simulink model "Lab05"  (R2024b)
settings: Solver=ode8  StartTime=0.0  StopTime=tf  FixedStep=0.025  RelTol=1e-3
values from neighbouring files (symbols this model uses):
  I = diag(Iv)    [initLab5.m]
  invI = inv(I)    [initLab5.m]
  w0 = [0.45; 0.52; 0.55]    [initLab5.m]
undefined symbols (not defined in the file or in its folder): IC
libraries: matrix_library x1
(part 3 of 4)

== system Lab05/EuleroCompletoCheGiraMaAlgebrico1/A313 ==
  In1 : Inport
  Cos : Trigonometry  Operator=cos
  Cos1 : Trigonometry  Operator=cos
  Cos2 : Trigonometry  Operator=cos
  Demux : Demux  Outputs=3
  Gain : Gain  Gain=-1
  Matrix Concatenate : Concatenate  NumInputs=3  Mode=Multidimensional array
  Matrix Concatenate1 : Concatenate  NumInputs=3  Mode=Multidimensional array
  Matrix Concatenate3 : Concatenate  NumInputs=3  Mode=Multidimensional array  ConcatenateDimension=2
  Matrix Concatenate4 : Concatenate  NumInputs=3  Mode=Multidimensional array
  Product{1,3,5..6,8,10..12} (8 alike) : Product
  Product{2,4,7,9} (4 alike) : Product  Inputs=3
  Sin : Trigonometry
  Sin1 : Trigonometry
  Sin2 : Trigonometry
  Subtract : Sum  Inputs=+-
  Subtract1 : Sum  Inputs=--
  Subtract2 : Sum
  Subtract3 : Sum  Inputs=-+
  Out1 : Outport
  wires:
  In1/1 -> Demux/1
  [cosTheta] -> Product2/3
  Product7/1 -> Subtract2/2
  [sinTheta] -> Product11/2
  [sinPhi] -> Product8/2
  Sin/1 -> [sinPhi]
  [cosTheta] -> Product4/3
  [sinPhi] -> Product2/2
  [sinTheta] -> Product10/2
  Product5/1 -> Matrix Concatenate/3
  [cosPsi] -> Product6/1
  Demux/3 -> Sin2/1, Cos2/1
  Product9/1 -> Subtract3/2
  [cosTheta] -> Matrix Concatenate1/3
  Matrix Concatenate1/1 -> Matrix Concatenate3/3
  [sinPsi] -> Product11/1
  Product2/1 -> Subtract/2
  [sinPhi] -> Product4/2
  Subtract2/1 -> Matrix Concatenate4/1
  Matrix Concatenate4/1 -> Matrix Concatenate3/2
  [cosPsi] -> Product12/1
  Cos2/1 -> [cosPsi]
  Product10/1 -> Gain/1
  [sinPsi] -> Product2/1
  [sinPsi] -> Product8/1
  Sin2/1 -> [sinPsi]
  [cosTheta] -> Product7/3
  Subtract/1 -> Matrix Concatenate/1
  [cosPhi] -> Product10/1
  Subtract1/1 -> Matrix Concatenate/2
  Subtract3/1 -> Matrix Concatenate4/2
  Demux/2 -> Sin1/1, Cos1/1
  [cosTheta] -> Product9/3
  Product8/1 -> Subtract3/1
  [cosPhi] -> Product9/2
  [cosPsi] -> Product9/1
  Gain/1 -> Matrix Concatenate4/3
  [cosPsi] -> Product4/1
  Product11/1 -> Matrix Concatenate1/1
  Product1/1 -> Subtract/1
  [cosPhi] -> Product1/2
  [sinTheta] -> Product12/2
  [cosPhi] -> Product7/2
  [sinPhi] -> Product6/2
  Product6/1 -> Subtract2/1
  Demux/1 -> Sin/1, Cos/1
  [cosPsi] -> Product1/1
  [sinPsi] -> Product7/1
  Cos1/1 -> [cosTheta]
  Sin1/1 -> [sinTheta]
  [sinTheta] -> Product5/2
  [sinPsi] -> Product3/1
  Product12/1 -> Matrix Concatenate1/2
  [sinPhi] -> Product5/1
  Product3/1 -> Subtract1/1
  Product4/1 -> Subtract1/2
  [cosPhi] -> Product3/2
  Matrix Concatenate/1 -> Matrix Concatenate3/1
  Cos/1 -> [cosPhi]
  Matrix Concatenate3/1 -> Out1/1

== system Lab05/EuleroCompletoCheGiraMaAlgebrico2/312 ==
  In1 : Inport
  In2 : Inport  Port=2
  In3 : Inport  Port=3
  Cos1 : Trigonometry  Operator=cos
  Cos2 : Trigonometry  Operator=cos
  Demux : Demux  Outputs=3
  Demux1 : Demux  Outputs=3
  Divide1 : Product  Inputs=*/
  IC : InitialCondition  Value=IC.angles
  Integrator1 : Integrator  ExternalReset=either  InitialConditionSource=external  WrapState=on  WrappedStateUpperValue=2*pi  WrappedStateLowerValue=0
  Integrator2 : Integrator  ExternalReset=either  InitialConditionSource=external  WrapState=on
  Integrator3 : Integrator  ExternalReset=either  InitialConditionSource=external  WrapState=on  WrappedStateUpperValue=2*pi  WrappedStateLowerValue=0
  Mux : Mux  Inputs=3
  Product{1..7} (7 alike) : Product
  Sin : Trigonometry
  Subtract : Sum  Inputs=+-
  Subtract1 : Sum
  Subtract2 : Sum  Inputs=+-
  Subtract3 : Sum  Inputs=+-
  Tan : Trigonometry  Operator=tan
  Out1 : Outport
  wires:
  Product6/1 -> Subtract3/2
  Product5/1 -> Subtract3/1
  Product4/1 -> Subtract1/2
  Integrator3/1 -> [theta3]
  [wz] -> Product5/1
  Mux/1 -> Out1/1
  Product7/1 -> Subtract2/2
  Cos1/1 -> [cosPsi]
  [theta3] -> Sin/1, Cos1/1
  [cosPsi] -> Product1/2
  Demux/2 -> [wy]
  Tan/1 -> [tanThe]
  Product2/1 -> Subtract/2
  [wz] -> Product3/1
  [tanThe] -> Product7/2
  Cos2/1 -> [cosThe]
  [cosPsi] -> Product5/2
  Divide1/1 -> Integrator1/1
  Subtract1/1 -> Integrator2/1
  Demux/3 -> [wz]
  [theta1] -> Mux/1
  Subtract/1 -> Divide1/1
  Demux/1 -> [wx]
  Subtract2/1 -> Integrator3/1
  [theta2] -> Tan/1, Cos2/1
  [wy] -> Subtract2/1
  Integrator1/1 -> [theta1]
  Integrator2/1 -> [theta2]
  [wx] -> Product4/1
  [sinPsi] -> Product2/2
  In1/1 -> Demux/1
  Subtract3/1 -> Product7/1
  Product3/1 -> Subtract1/1
  [theta2] -> Mux/2
  [sinPsi] -> Product3/2
  [theta3] -> Mux/3
  [sinPsi] -> Product6/2
  [wx] -> Product6/1
  [wx] -> Product2/1
  [cosPsi] -> Product4/2
  [wz] -> Product1/1
  Product1/1 -> Subtract/1
  [cosThe] -> Divide1/2
  Sin/1 -> [sinPsi]
  Demux1/1 -> Integrator1/3
  Demux1/2 -> Integrator2/3
  Demux1/3 -> Integrator3/3
  In2/1 -> IC/1
  IC/1 -> Demux1/1
  In3/1 -> Integrator2/2, Integrator3/2, Integrator1/2

== system Lab05/EuleroCompletoCheGiraMaAlgebrico2/312To313 ==
  note: Important
      |
      | This system is based on the assumptions that Phi and Psi ranges between [0 and 2*pi] while Theta ranges between [0 and pi]. This is consistent with 313 singularities
  note: Input Interface
  In1 : Inport
  Acos : Trigonometry  Operator=acos
  Acos1 : Trigonometry  Operator=acos
  Atan2 : Trigonometry  Operator=atan2
  Atan3 : Trigonometry  Operator=atan2
  Cos : Trigonometry  Operator=cos
  Cos1 : Trigonometry  Operator=cos
  Cos2 : Trigonometry  Operator=cos
  Demux : Demux  Outputs=3
  Divide{,1..3} (4 alike) : Product  Inputs=*/
  Gain : Gain  Gain=-1
  Gain1 : Gain  Gain=-1
  Mux : Mux  Inputs=3
  Product{,3,8,11} (4 alike) : Product
  Product4 : Product  Inputs=3
  Product9 : Product  Inputs=3
  Sin{,1..3} (4 alike) : Trigonometry
  Subtract1 : Sum
  Subtract3 : Sum  Inputs=+-
  Out1 : Outport
  wires:
  In1/1 -> Demux/1
  Mux/1 -> Out1/1
  Sin/1 -> [sinPhi312]
  Cos/1 -> [cosPhi312]
  Demux/1 -> Sin/1, Cos/1
  Sin1/1 -> [sinTheta312]
  Demux/2 -> Sin1/1, Cos1/1
  Cos1/1 -> [cosTheta312]
  Sin2/1 -> [sinPsi312]
  Cos2/1 -> [cosPsi312]
  Demux/3 -> Sin2/1, Cos2/1
  Product/1 -> Acos1/1, [cosTheta313]
  [cosTheta312] -> Product/2
  [cosPsi312] -> Product/1
  Atan2/1 -> Mux/1
  Acos/1 -> Mux/2
  Atan3/1 -> Mux/3
  [sinPhi313] -> Atan2/1
  [cosPhi313] -> Atan2/2
  [cosTheta313] -> Acos/1
  [cosPsi313] -> Atan3/2
  [sinPsi313] -> Atan3/1
  Sin3/1 -> [sinTheta313]
  Acos1/1 -> Sin3/1
  [cosPsi312] -> Product4/1
  [sinTheta312] -> Product4/3
  Product3/1 -> Subtract1/1
  [cosPhi312] -> Product3/2
  Product4/1 -> Subtract1/2
  [sinPsi312] -> Product3/1
  [sinPhi312] -> Product4/2
  Divide/1 -> [sinPhi313]
  [sinTheta313] -> Divide/2
  Subtract1/1 -> Divide/1
  Gain/1 -> [cosPhi313]
  Divide1/1 -> Gain/1
  [sinTheta313] -> Divide1/2
  [cosPsi312] -> Product9/1
  Product9/1 -> Subtract3/2
  Subtract3/1 -> Divide1/1
  [sinPsi312] -> Product8/1
  [cosPhi312] -> Product9/2
  [sinPhi312] -> Product8/2
  [sinTheta312] -> Product9/3
  Product8/1 -> Subtract3/1
  [sinTheta313] -> Divide2/2
  Divide2/1 -> [sinPsi313]
  [sinTheta313] -> Divide3/2
  Divide3/1 -> [cosPsi313]
  Product11/1 -> Gain1/1
  [sinPsi312] -> Product11/1
  [cosTheta312] -> Product11/2
  Gain1/1 -> Divide2/1
  [sinTheta312] -> Divide3/1

== system Lab05/EuleroCompletoCheGiraMaAlgebrico2/313 ==
  note: Phi
  note: Theta
  In2 : Inport
  In1 : Inport  Port=2
  In3 : Inport  Port=3
  Cos1 : Trigonometry  Operator=cos
  Cos2 : Trigonometry
  Demux : Demux  Outputs=3
  Demux1 : Demux  Outputs=3
  Divide : Product  Inputs=/
  Divide1 : Product  Inputs=*/
  IC : InitialCondition  Value=IC.angles
  Integrator1 : Integrator  ExternalReset=either  InitialConditionSource=external  WrapState=on  WrappedStateUpperValue=2*pi  WrappedStateLowerValue=0
  Integrator2 : Integrator  ExternalReset=either  InitialConditionSource=external  InitialCondition=pi/4  WrapState=on
  Integrator3 : Integrator  ExternalReset=either  InitialConditionSource=external  WrapState=on  WrappedStateUpperValue=2*pi  WrappedStateLowerValue=0
  Mux : Mux  Inputs=3
  Product{1..7} (7 alike) : Product
  Sin : Trigonometry
  Subtract : Sum
  Subtract1 : Sum  Inputs=-+
  Subtract2 : Sum  Inputs=+-
  Subtract3 : Sum
  Tan : Trigonometry  Operator=tan
  Out1 : Outport
  wires:
  [sinThe] -> Divide1/2
  Sin/1 -> [sinPsi]
  [wx] -> Product2/1
  [theta3] -> Mux/3
  [theta2] -> Mux/2
  Product3/1 -> Subtract1/1
  In1/1 -> Demux/1
  [sinPsi] -> Product3/2
  [sinPsi] -> Product6/2
  Subtract3/1 -> Product7/1
  Product1/1 -> Subtract/1
  [wx] -> Product6/1
  [wy] -> Product1/1
  [wz] -> Subtract2/1
  Subtract2/1 -> Integrator3/1
  [theta2] -> Tan/1, Cos2/1
  [cosPsi] -> Product4/2
  Demux/1 -> [wx]
  [sinPsi] -> Product2/2
  Integrator2/1 -> [theta2]
  [wx] -> Product4/1
  Tan/1 -> Divide/1
  [cosPsi] -> Product1/2
  Divide1/1 -> Integrator1/1
  Integrator1/1 -> [theta1]
  [ctanThe] -> Product7/2
  [cosPsi] -> Product5/2
  [wy] -> Product3/1
  Product2/1 -> Subtract/2
  Demux/2 -> [wy]
  Product5/1 -> Subtract3/1
  [wy] -> Product5/1
  Integrator3/1 -> [theta3]
  Product6/1 -> Subtract3/2
  Mux/1 -> Out1/1
  Product4/1 -> Subtract1/2
  [theta3] -> Sin/1, Cos1/1
  Product7/1 -> Subtract2/2
  Cos2/1 -> [sinThe]
  Subtract1/1 -> Integrator2/1
  [theta1] -> Mux/1
  Subtract/1 -> Divide1/1
  Demux/3 -> [wz]
  Cos1/1 -> [cosPsi]
  Divide/1 -> [ctanThe]
  Demux1/3 -> Integrator3/3
  Demux1/2 -> Integrator2/3
  Demux1/1 -> Integrator1/3
  IC/1 -> Demux1/1
  In3/1 -> Integrator1/2, Integrator2/2, Integrator3/2
  In2/1 -> IC/1

== system Lab05/EuleroCompletoCheGiraMaAlgebrico2/313To1 ==
  note: Input Interface
  note: Important
      |
      | This system is based on the assumptions that Phi and Psi ranges between [0 and 2*pi] while Theta ranges between [-pi/2 and pi/2]. This is consistent with 312 singularities
  In1 : Inport
  Acos : Trigonometry  Operator=asin
  Acos1 : Trigonometry  Operator=asin
  Atan2 : Trigonometry  Operator=atan2
  Atan3 : Trigonometry  Operator=atan2
  Cos : Trigonometry  Operator=cos
  Cos1 : Trigonometry  Operator=cos
  Cos2 : Trigonometry  Operator=cos
  Demux : Demux  Outputs=3
  Divide{,1..3} (4 alike) : Product  Inputs=*/
  Gain : Gain  Gain=-1
  Gain1 : Gain  Gain=-1
  Mux : Mux  Inputs=3
  Product{,3,8,11} (4 alike) : Product
  Product4 : Product  Inputs=3
  Product9 : Product  Inputs=3
  Sin : Trigonometry
  Sin1 : Trigonometry
  Sin2 : Trigonometry
  Sin3 : Trigonometry  Operator=cos
  Subtract1 : Sum  Inputs=--
  Subtract3 : Sum  Inputs=-+
  Out1 : Outport
  wires:
  Cos/1 -> [cosPhi313]
  Sin/1 -> [sinPhi313]
  Cos1/1 -> [cosTheta313]
  Demux/3 -> Sin2/1, Cos2/1
  Demux/1 -> Sin/1, Cos/1
  Sin2/1 -> [sinPsi313]
  Sin1/1 -> [sinTheta313]
  In1/1 -> Demux/1
  Demux/2 -> Sin1/1, Cos1/1
  Cos2/1 -> [cosPsi313]
  Mux/1 -> Out1/1
  [sinTheta312] -> Acos/1
  Atan3/1 -> Mux/3
  Atan2/1 -> Mux/1
  [sinPhi312] -> Atan2/1
  [cosPhi312] -> Atan2/2
  [sinPsi312] -> Atan3/1
  [cosPsi312] -> Atan3/2
  Acos/1 -> Mux/2
  [sinTheta313] -> Product/2
  Product/1 -> Acos1/1, [sinTheta312]
  Sin3/1 -> [cosTheta312]
  [cosPsi313] -> Product/1
  Acos1/1 -> Sin3/1
  Gain/1 -> [sinPhi312]
  Divide/1 -> Gain/1
  [cosTheta312] -> Divide/2
  Product3/1 -> Subtract1/1
  [cosPhi313] -> Product3/2
  Product4/1 -> Subtract1/2
  [cosPsi313] -> Product4/1
  [sinPhi313] -> Product4/2
  Subtract1/1 -> Divide/1
  [sinPsi313] -> Product3/1
  [cosTheta313] -> Product4/3
  [cosTheta312] -> Divide1/2
  Divide1/1 -> [cosPhi312]
  [cosPsi313] -> Product9/1
  Product9/1 -> Subtract3/2
  [sinPsi313] -> Product8/1
  [sinPhi313] -> Product8/2
  Product8/1 -> Subtract3/1
  [cosTheta313] -> Product9/3
  Subtract3/1 -> Divide1/1
  [cosPhi313] -> Product9/2
  Divide2/1 -> Gain1/1
  [cosTheta312] -> Divide2/2
  Gain1/1 -> [sinPsi312]
  [sinTheta313] -> Product11/2
  Product11/1 -> Divide2/1
  [sinPsi313] -> Product11/1
  [cosTheta312] -> Divide3/2
  [cosTheta313] -> Divide3/1
  Divide3/1 -> [cosPsi312]

== system Lab05/EuleroCompletoCheGiraMaAlgebrico2/313To312 ==
  note: Input Interface
  note: Important
      |
      | This system is based on the assumptions that Phi and Psi ranges between [0 and 2*pi] while Theta ranges between [-pi/2 and pi/2]. This is consistent with 312 singularities
  In1 : Inport
  Acos : Trigonometry  Operator=asin
  Acos1 : Trigonometry  Operator=asin
  Atan2 : Trigonometry  Operator=atan2
  Atan3 : Trigonometry  Operator=atan2
  Cos : Trigonometry  Operator=cos
  Cos1 : Trigonometry  Operator=cos
  Cos2 : Trigonometry  Operator=cos
  Demux : Demux  Outputs=3
  Divide{,1..3} (4 alike) : Product  Inputs=*/
  Gain : Gain  Gain=-1
  Gain1 : Gain  Gain=-1
  Mux : Mux  Inputs=3
  Product{,3,8,11} (4 alike) : Product
  Product4 : Product  Inputs=3
  Product9 : Product  Inputs=3
  Sin : Trigonometry
  Sin1 : Trigonometry
  Sin2 : Trigonometry
  Sin3 : Trigonometry  Operator=cos
  Subtract1 : Sum  Inputs=--
  Subtract3 : Sum  Inputs=-+
  Out1 : Outport
  wires:
  Cos/1 -> [cosPhi313]
  Sin/1 -> [sinPhi313]
  Cos1/1 -> [cosTheta313]
  Demux/3 -> Sin2/1, Cos2/1
  Demux/1 -> Sin/1, Cos/1
  Sin2/1 -> [sinPsi313]
  Sin1/1 -> [sinTheta313]
  In1/1 -> Demux/1
  Demux/2 -> Sin1/1, Cos1/1
  Cos2/1 -> [cosPsi313]
  Mux/1 -> Out1/1
  [sinTheta312] -> Acos/1
  Atan3/1 -> Mux/3
  Atan2/1 -> Mux/1
  [sinPhi312] -> Atan2/1
  [cosPhi312] -> Atan2/2
  [sinPsi312] -> Atan3/1
  [cosPsi312] -> Atan3/2
  Acos/1 -> Mux/2
  [sinTheta313] -> Product/2
  Product/1 -> Acos1/1, [sinTheta312]
  Sin3/1 -> [cosTheta312]
  [cosPsi313] -> Product/1
  Acos1/1 -> Sin3/1
  Gain/1 -> [sinPhi312]
  Divide/1 -> Gain/1
  [cosTheta312] -> Divide/2
  Product3/1 -> Subtract1/1
  [cosPhi313] -> Product3/2
  Product4/1 -> Subtract1/2
  [cosPsi313] -> Product4/1
  [sinPhi313] -> Product4/2
  Subtract1/1 -> Divide/1
  [sinPsi313] -> Product3/1
  [cosTheta313] -> Product4/3
  [cosTheta312] -> Divide1/2
  Divide1/1 -> [cosPhi312]
  [cosPsi313] -> Product9/1
  Product9/1 -> Subtract3/2
  [sinPsi313] -> Product8/1
  [sinPhi313] -> Product8/2
  Product8/1 -> Subtract3/1
  [cosTheta313] -> Product9/3
  Subtract3/1 -> Divide1/1
  [cosPhi313] -> Product9/2
  Divide2/1 -> Gain1/1
  [cosTheta312] -> Divide2/2
  Gain1/1 -> [sinPsi312]
  [sinTheta313] -> Product11/2
  Product11/1 -> Divide2/1
  [sinPsi313] -> Product11/1
  [cosTheta312] -> Divide3/2
  [cosTheta313] -> Divide3/1
  Divide3/1 -> [cosPsi312]

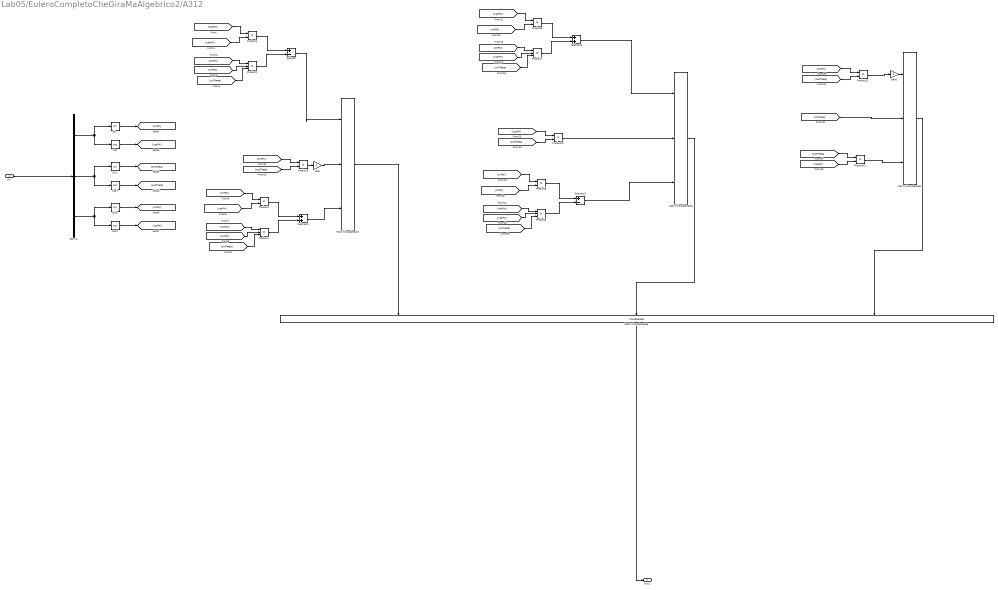
== system Lab05/EuleroCompletoCheGiraMaAlgebrico2/A312 ==
  In1 : Inport
  Cos : Trigonometry  Operator=cos
  Cos1 : Trigonometry  Operator=cos
  Cos2 : Trigonometry  Operator=cos
  Demux : Demux  Outputs=3
  Gain : Gain  Gain=-1
  Gain1 : Gain  Gain=-1
  Matrix Concatenate : Concatenate  NumInputs=3  Mode=Multidimensional array
  Matrix Concatenate1 : Concatenate  NumInputs=3  Mode=Multidimensional array
  Matrix Concatenate3 : Concatenate  NumInputs=3  Mode=Multidimensional array  ConcatenateDimension=2
  Matrix Concatenate4 : Concatenate  NumInputs=3  Mode=Multidimensional array
  Product{1,3,5..6,8,10..12} (8 alike) : Product
  Product{2,4,7,9} (4 alike) : Product  Inputs=3
  Sin : Trigonometry
  Sin1 : Trigonometry
  Sin2 : Trigonometry
  Subtract : Sum  Inputs=+-
  Subtract1 : Sum
  Subtract2 : Sum
  Subtract3 : Sum  Inputs=+-
  Out1 : Outport
  wires:
  In1/1 -> Demux/1
  [sinTheta] -> Product2/3
  Product7/1 -> Subtract2/2
  [cosTheta] -> Product11/2
  [sinPhi] -> Product8/2
  Sin/1 -> [sinPhi]
  [sinPhi] -> Product2/2
  [cosTheta] -> Product10/2
  [cosPsi] -> Product6/1
  Demux/3 -> Sin2/1, Cos2/1
  Product9/1 -> Subtract3/2
  [sinTheta] -> Matrix Concatenate1/2
  Matrix Concatenate1/1 -> Matrix Concatenate3/3
  [sinPsi] -> Product11/1
  Product2/1 -> Subtract/2
  Subtract2/1 -> Matrix Concatenate4/1
  Matrix Concatenate4/1 -> Matrix Concatenate3/2
  [cosTheta] -> Product12/1
  Cos2/1 -> [cosPsi]
  [sinPsi] -> Product2/1
  [sinPsi] -> Product8/1
  Sin2/1 -> [sinPsi]
  [sinTheta] -> Product7/3
  Subtract/1 -> Matrix Concatenate/1
  [cosPhi] -> Product10/1
  Demux/2 -> Sin1/1, Cos1/1
  [sinTheta] -> Product9/3
  Product8/1 -> Subtract3/1
  [cosPhi] -> Product9/2
  [cosPsi] -> Product9/1
  Product11/1 -> Gain1/1
  Product1/1 -> Subtract/1
  [cosPhi] -> Product1/2
  [cosPsi] -> Product12/2
  [cosPhi] -> Product7/2
  [sinPhi] -> Product6/2
  Product6/1 -> Subtract2/1
  Demux/1 -> Sin/1, Cos/1
  [cosPsi] -> Product1/1
  [sinPsi] -> Product7/1
  Cos1/1 -> [cosTheta]
  Sin1/1 -> [sinTheta]
  Product12/1 -> Matrix Concatenate1/3
  Matrix Concatenate/1 -> Matrix Concatenate3/1
  Cos/1 -> [cosPhi]
  Matrix Concatenate3/1 -> Out1/1
  Gain1/1 -> Matrix Concatenate1/1
  Product10/1 -> Matrix Concatenate4/2
  Subtract3/1 -> Matrix Concatenate4/3
  [cosPsi] -> Product4/1
  Product4/1 -> Subtract1/2
  [cosPhi] -> Product3/2
  Product3/1 -> Subtract1/1
  [sinPsi] -> Product3/1
  [sinPhi] -> Product4/2
  [sinTheta] -> Product4/3
  [sinPhi] -> Product5/1
  [cosTheta] -> Product5/2
  Product5/1 -> Gain/1
  Subtract1/1 -> Matrix Concatenate/3
  Gain/1 -> Matrix Concatenate/2

== system Lab05/EuleroCompletoCheGiraMaAlgebrico2/A313 ==
  In1 : Inport
  Cos : Trigonometry  Operator=cos
  Cos1 : Trigonometry  Operator=cos
  Cos2 : Trigonometry  Operator=cos
  Demux : Demux  Outputs=3
  Gain : Gain  Gain=-1
  Matrix Concatenate : Concatenate  NumInputs=3  Mode=Multidimensional array
  Matrix Concatenate1 : Concatenate  NumInputs=3  Mode=Multidimensional array
  Matrix Concatenate3 : Concatenate  NumInputs=3  Mode=Multidimensional array  ConcatenateDimension=2
  Matrix Concatenate4 : Concatenate  NumInputs=3  Mode=Multidimensional array
  Product{1,3,5..6,8,10..12} (8 alike) : Product
  Product{2,4,7,9} (4 alike) : Product  Inputs=3
  Sin : Trigonometry
  Sin1 : Trigonometry
  Sin2 : Trigonometry
  Subtract : Sum  Inputs=+-
  Subtract1 : Sum  Inputs=--
  Subtract2 : Sum
  Subtract3 : Sum  Inputs=-+
  Out1 : Outport
  wires:
  In1/1 -> Demux/1
  [cosTheta] -> Product2/3
  Product7/1 -> Subtract2/2
  [sinTheta] -> Product11/2
  [sinPhi] -> Product8/2
  Sin/1 -> [sinPhi]
  [cosTheta] -> Product4/3
  [sinPhi] -> Product2/2
  [sinTheta] -> Product10/2
  Product5/1 -> Matrix Concatenate/3
  [cosPsi] -> Product6/1
  Demux/3 -> Sin2/1, Cos2/1
  Product9/1 -> Subtract3/2
  [cosTheta] -> Matrix Concatenate1/3
  Matrix Concatenate1/1 -> Matrix Concatenate3/3
  [sinPsi] -> Product11/1
  Product2/1 -> Subtract/2
  [sinPhi] -> Product4/2
  Subtract2/1 -> Matrix Concatenate4/1
  Matrix Concatenate4/1 -> Matrix Concatenate3/2
  [cosPsi] -> Product12/1
  Cos2/1 -> [cosPsi]
  Product10/1 -> Gain/1
  [sinPsi] -> Product2/1
  [sinPsi] -> Product8/1
  Sin2/1 -> [sinPsi]
  [cosTheta] -> Product7/3
  Subtract/1 -> Matrix Concatenate/1
  [cosPhi] -> Product10/1
  Subtract1/1 -> Matrix Concatenate/2
  Subtract3/1 -> Matrix Concatenate4/2
  Demux/2 -> Sin1/1, Cos1/1
  [cosTheta] -> Product9/3
  Product8/1 -> Subtract3/1
  [cosPhi] -> Product9/2
  [cosPsi] -> Product9/1
  Gain/1 -> Matrix Concatenate4/3
  [cosPsi] -> Product4/1
  Product11/1 -> Matrix Concatenate1/1
  Product1/1 -> Subtract/1
  [cosPhi] -> Product1/2
  [sinTheta] -> Product12/2
  [cosPhi] -> Product7/2
  [sinPhi] -> Product6/2
  Product6/1 -> Subtract2/1
  Demux/1 -> Sin/1, Cos/1
  [cosPsi] -> Product1/1
  [sinPsi] -> Product7/1
  Cos1/1 -> [cosTheta]
  Sin1/1 -> [sinTheta]
  [sinTheta] -> Product5/2
  [sinPsi] -> Product3/1
  Product12/1 -> Matrix Concatenate1/2
  [sinPhi] -> Product5/1
  Product3/1 -> Subtract1/1
  Product4/1 -> Subtract1/2
  [cosPhi] -> Product3/2
  Matrix Concatenate/1 -> Matrix Concatenate3/1
  Cos/1 -> [cosPhi]
  Matrix Concatenate3/1 -> Out1/1

== system Lab05/EuleroCompletoCheGiraMale/312 ==
  In1 : Inport
  In2 : Inport  Port=2
  Enable : EnablePort  StatesWhenEnabling=reset
  Cos1 : Trigonometry  Operator=cos
  Cos2 : Trigonometry  Operator=cos
  Demux : Demux  Outputs=3
  Demux1 : Demux  Outputs=3
  Divide1 : Product  Inputs=*/
  IC : InitialCondition  Value=IC.angles
  Integrator1 : Integrator  InitialConditionSource=external  WrapState=on  WrappedStateUpperValue=2*pi  WrappedStateLowerValue=0
  Integrator2 : Integrator  InitialConditionSource=external  WrapState=on
  Integrator3 : Integrator  InitialConditionSource=external  WrapState=on  WrappedStateUpperValue=2*pi  WrappedStateLowerValue=0
  Mux : Mux  Inputs=3
  Product{1..7} (7 alike) : Product
  Sin : Trigonometry
  Subtract : Sum  Inputs=+-
  Subtract1 : Sum
  Subtract2 : Sum  Inputs=+-
  Subtract3 : Sum  Inputs=+-
  Tan : Trigonometry  Operator=tan
  Out1 : Outport
  wires:
  Product6/1 -> Subtract3/2
  Product5/1 -> Subtract3/1
  Product4/1 -> Subtract1/2
  Integrator3/1 -> [theta3]
  [wz] -> Product5/1
  Mux/1 -> Out1/1
  Product7/1 -> Subtract2/2
  Cos1/1 -> [cosPsi]
  [theta3] -> Sin/1, Cos1/1
  [cosPsi] -> Product1/2
  Demux/2 -> [wy]
  Tan/1 -> [tanThe]
  Product2/1 -> Subtract/2
  [wz] -> Product3/1
  [tanThe] -> Product7/2
  Cos2/1 -> [cosThe]
  [cosPsi] -> Product5/2
  Divide1/1 -> Integrator1/1
  Subtract1/1 -> Integrator2/1
  Demux/3 -> [wz]
  [theta1] -> Mux/1
  Subtract/1 -> Divide1/1
  Demux/1 -> [wx]
  Subtract2/1 -> Integrator3/1
  [theta2] -> Tan/1, Cos2/1
  [wy] -> Subtract2/1
  Integrator1/1 -> [theta1]
  Integrator2/1 -> [theta2]
  [wx] -> Product4/1
  [sinPsi] -> Product2/2
  In1/1 -> Demux/1
  Subtract3/1 -> Product7/1
  Product3/1 -> Subtract1/1
  [theta2] -> Mux/2
  [sinPsi] -> Product3/2
  [theta3] -> Mux/3
  [sinPsi] -> Product6/2
  [wx] -> Product6/1
  [wx] -> Product2/1
  [cosPsi] -> Product4/2
  [wz] -> Product1/1
  Product1/1 -> Subtract/1
  [cosThe] -> Divide1/2
  Sin/1 -> [sinPsi]
  Demux1/1 -> Integrator1/2
  Demux1/2 -> Integrator2/2
  Demux1/3 -> Integrator3/2
  In2/1 -> IC/1
  IC/1 -> Demux1/1

== system Lab05/EuleroCompletoCheGiraMale/312To313 ==
  note: Important
      |
      | This system is based on the assumptions that Phi and Psi ranges between [0 and 2*pi] while Theta ranges between [0 and pi]. This is consistent with 313 singularities
  note: Input Interface
  In1 : Inport
  Acos : Trigonometry  Operator=acos
  Acos1 : Trigonometry  Operator=acos
  Atan2 : Trigonometry  Operator=atan2
  Atan3 : Trigonometry  Operator=atan2
  Cos : Trigonometry  Operator=cos
  Cos1 : Trigonometry  Operator=cos
  Cos2 : Trigonometry  Operator=cos
  Demux : Demux  Outputs=3
  Divide{,1..3} (4 alike) : Product  Inputs=*/
  Gain : Gain  Gain=-1
  Gain1 : Gain  Gain=-1
  Mux : Mux  Inputs=3
  Product{,3,8,11} (4 alike) : Product
  Product4 : Product  Inputs=3
  Product9 : Product  Inputs=3
  Sin{,1..3} (4 alike) : Trigonometry
  Subtract1 : Sum
  Subtract3 : Sum  Inputs=+-
  Out1 : Outport
  wires:
  In1/1 -> Demux/1
  Mux/1 -> Out1/1
  Sin/1 -> [sinPhi312]
  Cos/1 -> [cosPhi312]
  Demux/1 -> Sin/1, Cos/1
  Sin1/1 -> [sinTheta312]
  Demux/2 -> Sin1/1, Cos1/1
  Cos1/1 -> [cosTheta312]
  Sin2/1 -> [sinPsi312]
  Cos2/1 -> [cosPsi312]
  Demux/3 -> Sin2/1, Cos2/1
  Product/1 -> Acos1/1, [cosTheta313]
  [cosTheta312] -> Product/2
  [cosPsi312] -> Product/1
  Atan2/1 -> Mux/1
  Acos/1 -> Mux/2
  Atan3/1 -> Mux/3
  [sinPhi313] -> Atan2/1
  [cosPhi313] -> Atan2/2
  [cosTheta313] -> Acos/1
  [cosPsi313] -> Atan3/2
  [sinPsi313] -> Atan3/1
  Sin3/1 -> [sinTheta313]
  Acos1/1 -> Sin3/1
  [cosPsi312] -> Product4/1
  [sinTheta312] -> Product4/3
  Product3/1 -> Subtract1/1
  [cosPhi312] -> Product3/2
  Product4/1 -> Subtract1/2
  [sinPsi312] -> Product3/1
  [sinPhi312] -> Product4/2
  Divide/1 -> [sinPhi313]
  [sinTheta313] -> Divide/2
  Subtract1/1 -> Divide/1
  Gain/1 -> [cosPhi313]
  Divide1/1 -> Gain/1
  [sinTheta313] -> Divide1/2
  [cosPsi312] -> Product9/1
  Product9/1 -> Subtract3/2
  Subtract3/1 -> Divide1/1
  [sinPsi312] -> Product8/1
  [cosPhi312] -> Product9/2
  [sinPhi312] -> Product8/2
  [sinTheta312] -> Product9/3
  Product8/1 -> Subtract3/1
  [sinTheta313] -> Divide2/2
  Divide2/1 -> [sinPsi313]
  [sinTheta313] -> Divide3/2
  Divide3/1 -> [cosPsi313]
  Product11/1 -> Gain1/1
  [sinPsi312] -> Product11/1
  [cosTheta312] -> Product11/2
  Gain1/1 -> Divide2/1
  [sinTheta312] -> Divide3/1

== system Lab05/EuleroCompletoCheGiraMale/313 ==
  note: Phi
  note: Theta
  In2 : Inport
  In1 : Inport  Port=2
  Enable : EnablePort  StatesWhenEnabling=reset
  Cos1 : Trigonometry  Operator=cos
  Cos2 : Trigonometry
  Demux : Demux  Outputs=3
  Demux1 : Demux  Outputs=3
  Divide : Product  Inputs=/
  Divide1 : Product  Inputs=*/
  IC : InitialCondition  Value=IC.angles
  Integrator1 : Integrator  InitialConditionSource=external  WrapState=on  WrappedStateUpperValue=2*pi  WrappedStateLowerValue=0
  Integrator2 : Integrator  InitialConditionSource=external  InitialCondition=pi/4  WrapState=on
  Integrator3 : Integrator  InitialConditionSource=external  WrapState=on  WrappedStateUpperValue=2*pi  WrappedStateLowerValue=0
  Mux : Mux  Inputs=3
  Product{1..7} (7 alike) : Product
  Sin : Trigonometry
  Subtract : Sum
  Subtract1 : Sum  Inputs=-+
  Subtract2 : Sum  Inputs=+-
  Subtract3 : Sum
  Tan : Trigonometry  Operator=tan
  Out1 : Outport
  wires:
  [sinThe] -> Divide1/2
  Sin/1 -> [sinPsi]
  [wx] -> Product2/1
  [theta3] -> Mux/3
  [theta2] -> Mux/2
  Product3/1 -> Subtract1/1
  In1/1 -> Demux/1
  [sinPsi] -> Product3/2
  [sinPsi] -> Product6/2
  Subtract3/1 -> Product7/1
  Product1/1 -> Subtract/1
  [wx] -> Product6/1
  [wy] -> Product1/1
  [wz] -> Subtract2/1
  Subtract2/1 -> Integrator3/1
  [theta2] -> Tan/1, Cos2/1
  [cosPsi] -> Product4/2
  Demux/1 -> [wx]
  [sinPsi] -> Product2/2
  Integrator2/1 -> [theta2]
  [wx] -> Product4/1
  Tan/1 -> Divide/1
  [cosPsi] -> Product1/2
  Divide1/1 -> Integrator1/1
  Integrator1/1 -> [theta1]
  [ctanThe] -> Product7/2
  [cosPsi] -> Product5/2
  [wy] -> Product3/1
  Product2/1 -> Subtract/2
  Demux/2 -> [wy]
  Product5/1 -> Subtract3/1
  [wy] -> Product5/1
  Integrator3/1 -> [theta3]
  Product6/1 -> Subtract3/2
  Mux/1 -> Out1/1
  Product4/1 -> Subtract1/2
  [theta3] -> Sin/1, Cos1/1
  Product7/1 -> Subtract2/2
  Cos2/1 -> [sinThe]
  Subtract1/1 -> Integrator2/1
  [theta1] -> Mux/1
  Subtract/1 -> Divide1/1
  Demux/3 -> [wz]
  Cos1/1 -> [cosPsi]
  Divide/1 -> [ctanThe]
  Demux1/3 -> Integrator3/2
  Demux1/2 -> Integrator2/2
  Demux1/1 -> Integrator1/2
  In2/1 -> IC/1
  IC/1 -> Demux1/1

== system Lab05/EuleroCompletoCheGiraMale/313To1 ==
  note: Input Interface
  note: Important
      |
      | This system is based on the assumptions that Phi and Psi ranges between [0 and 2*pi] while Theta ranges between [-pi/2 and pi/2]. This is consistent with 312 singularities
  In1 : Inport
  Acos : Trigonometry  Operator=asin
  Acos1 : Trigonometry  Operator=asin
  Atan2 : Trigonometry  Operator=atan2
  Atan3 : Trigonometry  Operator=atan2
  Cos : Trigonometry  Operator=cos
  Cos1 : Trigonometry  Operator=cos
  Cos2 : Trigonometry  Operator=cos
  Demux : Demux  Outputs=3
  Divide{,1..3} (4 alike) : Product  Inputs=*/
  Gain : Gain  Gain=-1
  Gain1 : Gain  Gain=-1
  Mux : Mux  Inputs=3
  Product{,3,8,11} (4 alike) : Product
  Product4 : Product  Inputs=3
  Product9 : Product  Inputs=3
  Sin : Trigonometry
  Sin1 : Trigonometry
  Sin2 : Trigonometry
  Sin3 : Trigonometry  Operator=cos
  Subtract1 : Sum  Inputs=--
  Subtract3 : Sum  Inputs=-+
  Out1 : Outport
  wires:
  Cos/1 -> [cosPhi313]
  Sin/1 -> [sinPhi313]
  Cos1/1 -> [cosTheta313]
  Demux/3 -> Sin2/1, Cos2/1
  Demux/1 -> Sin/1, Cos/1
  Sin2/1 -> [sinPsi313]
  Sin1/1 -> [sinTheta313]
  In1/1 -> Demux/1
  Demux/2 -> Sin1/1, Cos1/1
  Cos2/1 -> [cosPsi313]
  Mux/1 -> Out1/1
  [sinTheta312] -> Acos/1
  Atan3/1 -> Mux/3
  Atan2/1 -> Mux/1
  [sinPhi312] -> Atan2/1
  [cosPhi312] -> Atan2/2
  [sinPsi312] -> Atan3/1
  [cosPsi312] -> Atan3/2
  Acos/1 -> Mux/2
  [sinTheta313] -> Product/2
  Product/1 -> Acos1/1, [sinTheta312]
  Sin3/1 -> [cosTheta312]
  [cosPsi313] -> Product/1
  Acos1/1 -> Sin3/1
  Gain/1 -> [sinPhi312]
  Divide/1 -> Gain/1
  [cosTheta312] -> Divide/2
  Product3/1 -> Subtract1/1
  [cosPhi313] -> Product3/2
  Product4/1 -> Subtract1/2
  [cosPsi313] -> Product4/1
  [sinPhi313] -> Product4/2
  Subtract1/1 -> Divide/1
  [sinPsi313] -> Product3/1
  [cosTheta313] -> Product4/3
  [cosTheta312] -> Divide1/2
  Divide1/1 -> [cosPhi312]
  [cosPsi313] -> Product9/1
  Product9/1 -> Subtract3/2
  [sinPsi313] -> Product8/1
  [sinPhi313] -> Product8/2
  Product8/1 -> Subtract3/1
  [cosTheta313] -> Product9/3
  Subtract3/1 -> Divide1/1
  [cosPhi313] -> Product9/2
  Divide2/1 -> Gain1/1
  [cosTheta312] -> Divide2/2
  Gain1/1 -> [sinPsi312]
  [sinTheta313] -> Product11/2
  Product11/1 -> Divide2/1
  [sinPsi313] -> Product11/1
  [cosTheta312] -> Divide3/2
  [cosTheta313] -> Divide3/1
  Divide3/1 -> [cosPsi312]

== system Lab05/EuleroCompletoCheGiraMale/313To312 ==
  note: Input Interface
  note: Important
      |
      | This system is based on the assumptions that Phi and Psi ranges between [0 and 2*pi] while Theta ranges between [-pi/2 and pi/2]. This is consistent with 312 singularities
  In1 : Inport
  Acos : Trigonometry  Operator=asin
  Acos1 : Trigonometry  Operator=asin
  Atan2 : Trigonometry  Operator=atan2
  Atan3 : Trigonometry  Operator=atan2
  Cos : Trigonometry  Operator=cos
  Cos1 : Trigonometry  Operator=cos
  Cos2 : Trigonometry  Operator=cos
  Demux : Demux  Outputs=3
  Divide{,1..3} (4 alike) : Product  Inputs=*/
  Gain : Gain  Gain=-1
  Gain1 : Gain  Gain=-1
  Mux : Mux  Inputs=3
  Product{,3,8,11} (4 alike) : Product
  Product4 : Product  Inputs=3
  Product9 : Product  Inputs=3
  Sin : Trigonometry
  Sin1 : Trigonometry
  Sin2 : Trigonometry
  Sin3 : Trigonometry  Operator=cos
  Subtract1 : Sum  Inputs=--
  Subtract3 : Sum  Inputs=-+
  Out1 : Outport
  wires:
  Cos/1 -> [cosPhi313]
  Sin/1 -> [sinPhi313]
  Cos1/1 -> [cosTheta313]
  Demux/3 -> Sin2/1, Cos2/1
  Demux/1 -> Sin/1, Cos/1
  Sin2/1 -> [sinPsi313]
  Sin1/1 -> [sinTheta313]
  In1/1 -> Demux/1
  Demux/2 -> Sin1/1, Cos1/1
  Cos2/1 -> [cosPsi313]
  Mux/1 -> Out1/1
  [sinTheta312] -> Acos/1
  Atan3/1 -> Mux/3
  Atan2/1 -> Mux/1
  [sinPhi312] -> Atan2/1
  [cosPhi312] -> Atan2/2
  [sinPsi312] -> Atan3/1
  [cosPsi312] -> Atan3/2
  Acos/1 -> Mux/2
  [sinTheta313] -> Product/2
  Product/1 -> Acos1/1, [sinTheta312]
  Sin3/1 -> [cosTheta312]
  [cosPsi313] -> Product/1
  Acos1/1 -> Sin3/1
  Gain/1 -> [sinPhi312]
  Divide/1 -> Gain/1
  [cosTheta312] -> Divide/2
  Product3/1 -> Subtract1/1
  [cosPhi313] -> Product3/2
  Product4/1 -> Subtract1/2
  [cosPsi313] -> Product4/1
  [sinPhi313] -> Product4/2
  Subtract1/1 -> Divide/1
  [sinPsi313] -> Product3/1
  [cosTheta313] -> Product4/3
  [cosTheta312] -> Divide1/2
  Divide1/1 -> [cosPhi312]
  [cosPsi313] -> Product9/1
  Product9/1 -> Subtract3/2
  [sinPsi313] -> Product8/1
  [sinPhi313] -> Product8/2
  Product8/1 -> Subtract3/1
  [cosTheta313] -> Product9/3
  Subtract3/1 -> Divide1/1
  [cosPhi313] -> Product9/2
  Divide2/1 -> Gain1/1
  [cosTheta312] -> Divide2/2
  Gain1/1 -> [sinPsi312]
  [sinTheta313] -> Product11/2
  Product11/1 -> Divide2/1
  [sinPsi313] -> Product11/1
  [cosTheta312] -> Divide3/2
  [cosTheta313] -> Divide3/1
  Divide3/1 -> [cosPsi312]

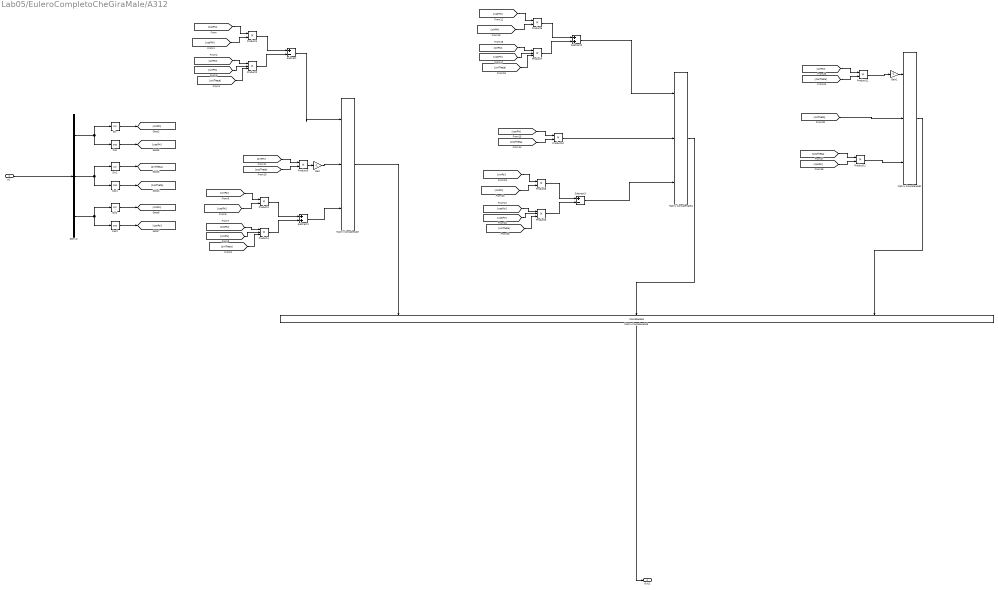
== system Lab05/EuleroCompletoCheGiraMale/A312 ==
  In1 : Inport
  Cos : Trigonometry  Operator=cos
  Cos1 : Trigonometry  Operator=cos
  Cos2 : Trigonometry  Operator=cos
  Demux : Demux  Outputs=3
  Gain : Gain  Gain=-1
  Gain1 : Gain  Gain=-1
  Matrix Concatenate : Concatenate  NumInputs=3  Mode=Multidimensional array
  Matrix Concatenate1 : Concatenate  NumInputs=3  Mode=Multidimensional array
  Matrix Concatenate3 : Concatenate  NumInputs=3  Mode=Multidimensional array  ConcatenateDimension=2
  Matrix Concatenate4 : Concatenate  NumInputs=3  Mode=Multidimensional array
  Product{1,3,5..6,8,10..12} (8 alike) : Product
  Product{2,4,7,9} (4 alike) : Product  Inputs=3
  Sin : Trigonometry
  Sin1 : Trigonometry
  Sin2 : Trigonometry
  Subtract : Sum  Inputs=+-
  Subtract1 : Sum
  Subtract2 : Sum
  Subtract3 : Sum  Inputs=+-
  Out1 : Outport
  wires:
  In1/1 -> Demux/1
  [sinTheta] -> Product2/3
  Product7/1 -> Subtract2/2
  [cosTheta] -> Product11/2
  [sinPhi] -> Product8/2
  Sin/1 -> [sinPhi]
  [sinPhi] -> Product2/2
  [cosTheta] -> Product10/2
  [cosPsi] -> Product6/1
  Demux/3 -> Sin2/1, Cos2/1
  Product9/1 -> Subtract3/2
  [sinTheta] -> Matrix Concatenate1/2
  Matrix Concatenate1/1 -> Matrix Concatenate3/3
  [sinPsi] -> Product11/1
  Product2/1 -> Subtract/2
  Subtract2/1 -> Matrix Concatenate4/1
  Matrix Concatenate4/1 -> Matrix Concatenate3/2
  [cosTheta] -> Product12/1
  Cos2/1 -> [cosPsi]
  [sinPsi] -> Product2/1
  [sinPsi] -> Product8/1
  Sin2/1 -> [sinPsi]
  [sinTheta] -> Product7/3
  Subtract/1 -> Matrix Concatenate/1
  [cosPhi] -> Product10/1
  Demux/2 -> Sin1/1, Cos1/1
  [sinTheta] -> Product9/3
  Product8/1 -> Subtract3/1
  [cosPhi] -> Product9/2
  [cosPsi] -> Product9/1
  Product11/1 -> Gain1/1
  Product1/1 -> Subtract/1
  [cosPhi] -> Product1/2
  [cosPsi] -> Product12/2
  [cosPhi] -> Product7/2
  [sinPhi] -> Product6/2
  Product6/1 -> Subtract2/1
  Demux/1 -> Sin/1, Cos/1
  [cosPsi] -> Product1/1
  [sinPsi] -> Product7/1
  Cos1/1 -> [cosTheta]
  Sin1/1 -> [sinTheta]
  Product12/1 -> Matrix Concatenate1/3
  Matrix Concatenate/1 -> Matrix Concatenate3/1
  Cos/1 -> [cosPhi]
  Matrix Concatenate3/1 -> Out1/1
  Gain1/1 -> Matrix Concatenate1/1
  Product10/1 -> Matrix Concatenate4/2
  Subtract3/1 -> Matrix Concatenate4/3
  [cosPsi] -> Product4/1
  Product4/1 -> Subtract1/2
  [cosPhi] -> Product3/2
  Product3/1 -> Subtract1/1
  [sinPsi] -> Product3/1
  [sinPhi] -> Product4/2
  [sinTheta] -> Product4/3
  [sinPhi] -> Product5/1
  [cosTheta] -> Product5/2
  Product5/1 -> Gain/1
  Subtract1/1 -> Matrix Concatenate/3
  Gain/1 -> Matrix Concatenate/2

== system Lab05/EuleroCompletoCheGiraMale/A313 ==
  In1 : Inport
  Cos : Trigonometry  Operator=cos
  Cos1 : Trigonometry  Operator=cos
  Cos2 : Trigonometry  Operator=cos
  Demux : Demux  Outputs=3
  Gain : Gain  Gain=-1
  Matrix Concatenate : Concatenate  NumInputs=3  Mode=Multidimensional array
  Matrix Concatenate1 : Concatenate  NumInputs=3  Mode=Multidimensional array
  Matrix Concatenate3 : Concatenate  NumInputs=3  Mode=Multidimensional array  ConcatenateDimension=2
  Matrix Concatenate4 : Concatenate  NumInputs=3  Mode=Multidimensional array
  Product{1,3,5..6,8,10..12} (8 alike) : Product
  Product{2,4,7,9} (4 alike) : Product  Inputs=3
  Sin : Trigonometry
  Sin1 : Trigonometry
  Sin2 : Trigonometry
  Subtract : Sum  Inputs=+-
  Subtract1 : Sum  Inputs=--
  Subtract2 : Sum
  Subtract3 : Sum  Inputs=-+
  Out1 : Outport
  wires:
  In1/1 -> Demux/1
  [cosTheta] -> Product2/3
  Product7/1 -> Subtract2/2
  [sinTheta] -> Product11/2
  [sinPhi] -> Product8/2
  Sin/1 -> [sinPhi]
  [cosTheta] -> Product4/3
  [sinPhi] -> Product2/2
  [sinTheta] -> Product10/2
  Product5/1 -> Matrix Concatenate/3
  [cosPsi] -> Product6/1
  Demux/3 -> Sin2/1, Cos2/1
  Product9/1 -> Subtract3/2
  [cosTheta] -> Matrix Concatenate1/3
  Matrix Concatenate1/1 -> Matrix Concatenate3/3
  [sinPsi] -> Product11/1
  Product2/1 -> Subtract/2
  [sinPhi] -> Product4/2
  Subtract2/1 -> Matrix Concatenate4/1
  Matrix Concatenate4/1 -> Matrix Concatenate3/2
  [cosPsi] -> Product12/1
  Cos2/1 -> [cosPsi]
  Product10/1 -> Gain/1
  [sinPsi] -> Product2/1
  [sinPsi] -> Product8/1
  Sin2/1 -> [sinPsi]
  [cosTheta] -> Product7/3
  Subtract/1 -> Matrix Concatenate/1
  [cosPhi] -> Product10/1
  Subtract1/1 -> Matrix Concatenate/2
  Subtract3/1 -> Matrix Concatenate4/2
  Demux/2 -> Sin1/1, Cos1/1
  [cosTheta] -> Product9/3
  Product8/1 -> Subtract3/1
  [cosPhi] -> Product9/2
  [cosPsi] -> Product9/1
  Gain/1 -> Matrix Concatenate4/3
  [cosPsi] -> Product4/1
  Product11/1 -> Matrix Concatenate1/1
  Product1/1 -> Subtract/1
  [cosPhi] -> Product1/2
  [sinTheta] -> Product12/2
  [cosPhi] -> Product7/2
  [sinPhi] -> Product6/2
  Product6/1 -> Subtract2/1
  Demux/1 -> Sin/1, Cos/1
  [cosPsi] -> Product1/1
  [sinPsi] -> Product7/1
  Cos1/1 -> [cosTheta]
  Sin1/1 -> [sinTheta]
  [sinTheta] -> Product5/2
  [sinPsi] -> Product3/1
  Product12/1 -> Matrix Concatenate1/2
  [sinPhi] -> Product5/1
  Product3/1 -> Subtract1/1
  Product4/1 -> Subtract1/2
  [cosPhi] -> Product3/2
  Matrix Concatenate/1 -> Matrix Concatenate3/1
  Cos/1 -> [cosPhi]
  Matrix Concatenate3/1 -> Out1/1

== system Lab05/Ordinato/312 ==
  In2 : Inport
  In1 : Inport  Port=2
  In3 : Inport  Port=3
  Cos1 : Trigonometry  Operator=cos
  Cos2 : Trigonometry  Operator=cos
  Demux : Demux  Outputs=3
  Demux1 : Demux  Outputs=3
  Divide1 : Product  Inputs=*/
  Integrator1 : Integrator  ExternalReset=either  InitialConditionSource=external  WrapState=on  WrappedStateUpperValue=2*pi  WrappedStateLowerValue=0
  Integrator2 : Integrator  ExternalReset=either  InitialConditionSource=external  WrapState=on
  Integrator3 : Integrator  ExternalReset=either  InitialConditionSource=external  WrapState=on  WrappedStateUpperValue=2*pi  WrappedStateLowerValue=0
  Mux : Mux  Inputs=3
  Product{1..7} (7 alike) : Product
  Sin : Trigonometry
  Subtract : Sum  Inputs=+-
  Subtract1 : Sum
  Subtract2 : Sum  Inputs=+-
  Subtract3 : Sum  Inputs=+-
  Tan : Trigonometry  Operator=tan
  Out1 : Outport
  wires:
  Product6/1 -> Subtract3/2
  Product5/1 -> Subtract3/1
  Product4/1 -> Subtract1/2
  Integrator3/1 -> [theta3]
  [wz] -> Product5/1
  Mux/1 -> Out1/1
  Product7/1 -> Subtract2/2
  Cos1/1 -> [cosPsi]
  [theta3] -> Sin/1, Cos1/1
  [cosPsi] -> Product1/2
  Demux/2 -> [wy]
  Tan/1 -> [tanThe]
  Product2/1 -> Subtract/2
  [wz] -> Product3/1
  [tanThe] -> Product7/2
  Cos2/1 -> [cosThe]
  [cosPsi] -> Product5/2
  Divide1/1 -> Integrator1/1
  Subtract1/1 -> Integrator2/1
  Demux/3 -> [wz]
  [theta1] -> Mux/1
  Subtract/1 -> Divide1/1
  Demux/1 -> [wx]
  Subtract2/1 -> Integrator3/1
  [theta2] -> Tan/1, Cos2/1
  [wy] -> Subtract2/1
  Integrator1/1 -> [theta1]
  Integrator2/1 -> [theta2]
  [wx] -> Product4/1
  [sinPsi] -> Product2/2
  In1/1 -> Demux/1
  Subtract3/1 -> Product7/1
  Product3/1 -> Subtract1/1
  [theta2] -> Mux/2
  [sinPsi] -> Product3/2
  [theta3] -> Mux/3
  [sinPsi] -> Product6/2
  [wx] -> Product6/1
  [wx] -> Product2/1
  [cosPsi] -> Product4/2
  [wz] -> Product1/1
  Product1/1 -> Subtract/1
  [cosThe] -> Divide1/2
  Sin/1 -> [sinPsi]
  Demux1/1 -> Integrator1/3
  Demux1/2 -> Integrator2/3
  Demux1/3 -> Integrator3/3
  In2/1 -> Demux1/1
  In3/1 -> Integrator2/2, Integrator3/2, Integrator1/2

== system Lab05/Ordinato/312To313 ==
  note: Important
      |
      | This system is based on the assumptions that Phi and Psi ranges between [0 and 2*pi] while Theta ranges between [0 and pi]. This is consistent with 313 singularities
  note: Input Interface
  In1 : Inport
  Acos : Trigonometry  Operator=acos
  Acos1 : Trigonometry  Operator=acos
  Atan2 : Trigonometry  Operator=atan2
  Atan3 : Trigonometry  Operator=atan2
  Cos : Trigonometry  Operator=cos
  Cos1 : Trigonometry  Operator=cos
  Cos2 : Trigonometry  Operator=cos
  Demux : Demux  Outputs=3
  Divide{,1..3} (4 alike) : Product  Inputs=*/
  Gain : Gain  Gain=-1
  Gain1 : Gain  Gain=-1
  Mux : Mux  Inputs=3
  Product{,3,8,11} (4 alike) : Product
  Product4 : Product  Inputs=3
  Product9 : Product  Inputs=3
  Sin{,1..3} (4 alike) : Trigonometry
  Subtract1 : Sum
  Subtract3 : Sum  Inputs=+-
  Out1 : Outport
  wires:
  In1/1 -> Demux/1
  Mux/1 -> Out1/1
  Sin/1 -> [sinPhi312]
  Cos/1 -> [cosPhi312]
  Demux/1 -> Sin/1, Cos/1
  Sin1/1 -> [sinTheta312]
  Demux/2 -> Sin1/1, Cos1/1
  Cos1/1 -> [cosTheta312]
  Sin2/1 -> [sinPsi312]
  Cos2/1 -> [cosPsi312]
  Demux/3 -> Sin2/1, Cos2/1
  Product/1 -> Acos1/1, [cosTheta313]
  [cosTheta312] -> Product/2
  [cosPsi312] -> Product/1
  Atan2/1 -> Mux/1
  Acos/1 -> Mux/2
  Atan3/1 -> Mux/3
  [sinPhi313] -> Atan2/1
  [cosPhi313] -> Atan2/2
  [cosTheta313] -> Acos/1
  [cosPsi313] -> Atan3/2
  [sinPsi313] -> Atan3/1
  Sin3/1 -> [sinTheta313]
  Acos1/1 -> Sin3/1
  [cosPsi312] -> Product4/1
  [sinTheta312] -> Product4/3
  Product3/1 -> Subtract1/1
  [cosPhi312] -> Product3/2
  Product4/1 -> Subtract1/2
  [sinPsi312] -> Product3/1
  [sinPhi312] -> Product4/2
  Divide/1 -> [sinPhi313]
  [sinTheta313] -> Divide/2
  Subtract1/1 -> Divide/1
  Gain/1 -> [cosPhi313]
  Divide1/1 -> Gain/1
  [sinTheta313] -> Divide1/2
  [cosPsi312] -> Product9/1
  Product9/1 -> Subtract3/2
  Subtract3/1 -> Divide1/1
  [sinPsi312] -> Product8/1
  [cosPhi312] -> Product9/2
  [sinPhi312] -> Product8/2
  [sinTheta312] -> Product9/3
  Product8/1 -> Subtract3/1
  [sinTheta313] -> Divide2/2
  Divide2/1 -> [sinPsi313]
  [sinTheta313] -> Divide3/2
  Divide3/1 -> [cosPsi313]
  Product11/1 -> Gain1/1
  [sinPsi312] -> Product11/1
  [cosTheta312] -> Product11/2
  Gain1/1 -> Divide2/1
  [sinTheta312] -> Divide3/1

== system Lab05/Ordinato/313 ==
  note: Phi
  note: Theta
  In3 : Inport
  In1 : Inport  Port=2
  In2 : Inport  Port=3
  Cos1 : Trigonometry  Operator=cos
  Cos2 : Trigonometry
  Demux : Demux  Outputs=3
  Demux1 : Demux  Outputs=3
  Divide : Product  Inputs=/
  Divide1 : Product  Inputs=*/
  Integrator1 : Integrator  ExternalReset=either  InitialConditionSource=external  WrapState=on  WrappedStateUpperValue=2*pi  WrappedStateLowerValue=0
  Integrator2 : Integrator  ExternalReset=either  InitialConditionSource=external  InitialCondition=pi/4  WrapState=on
  Integrator3 : Integrator  ExternalReset=either  InitialConditionSource=external  WrapState=on  WrappedStateUpperValue=2*pi  WrappedStateLowerValue=0
  Mux : Mux  Inputs=3
  Product{1..7} (7 alike) : Product
  Sin : Trigonometry
  Subtract : Sum
  Subtract1 : Sum  Inputs=-+
  Subtract2 : Sum  Inputs=+-
  Subtract3 : Sum
  Tan : Trigonometry  Operator=tan
  Out1 : Outport
  wires:
  [sinThe] -> Divide1/2
  Sin/1 -> [sinPsi]
  [wx] -> Product2/1
  [theta3] -> Mux/3
  [theta2] -> Mux/2
  Product3/1 -> Subtract1/1
  In1/1 -> Demux/1
  [sinPsi] -> Product3/2
  [sinPsi] -> Product6/2
  Subtract3/1 -> Product7/1
  Product1/1 -> Subtract/1
  [wx] -> Product6/1
  [wy] -> Product1/1
  [wz] -> Subtract2/1
  Subtract2/1 -> Integrator3/1
  [theta2] -> Tan/1, Cos2/1
  [cosPsi] -> Product4/2
  Demux/1 -> [wx]
  [sinPsi] -> Product2/2
  Integrator2/1 -> [theta2]
  [wx] -> Product4/1
  Tan/1 -> Divide/1
  [cosPsi] -> Product1/2
  Divide1/1 -> Integrator1/1
  Integrator1/1 -> [theta1]
  [ctanThe] -> Product7/2
  [cosPsi] -> Product5/2
  [wy] -> Product3/1
  Product2/1 -> Subtract/2
  Demux/2 -> [wy]
  Product5/1 -> Subtract3/1
  [wy] -> Product5/1
  Integrator3/1 -> [theta3]
  Product6/1 -> Subtract3/2
  Mux/1 -> Out1/1
  Product4/1 -> Subtract1/2
  [theta3] -> Sin/1, Cos1/1
  Product7/1 -> Subtract2/2
  Cos2/1 -> [sinThe]
  Subtract1/1 -> Integrator2/1
  [theta1] -> Mux/1
  Subtract/1 -> Divide1/1
  Demux/3 -> [wz]
  Cos1/1 -> [cosPsi]
  Divide/1 -> [ctanThe]
  Demux1/3 -> Integrator3/3
  Demux1/2 -> Integrator2/3
  Demux1/1 -> Integrator1/3
  In2/1 -> Demux1/1
  In3/1 -> Integrator1/2, Integrator2/2, Integrator3/2

== system Lab05/Ordinato/313To312 ==
  note: Input Interface
  note: Important
      |
      | This system is based on the assumptions that Phi and Psi ranges between [0 and 2*pi] while Theta ranges between [-pi/2 and pi/2]. This is consistent with 312 singularities
  In1 : Inport
  Acos : Trigonometry  Operator=asin
  Acos1 : Trigonometry  Operator=asin
  Atan2 : Trigonometry  Operator=atan2
  Atan3 : Trigonometry  Operator=atan2
  Cos : Trigonometry  Operator=cos
  Cos1 : Trigonometry  Operator=cos
  Cos2 : Trigonometry  Operator=cos
  Demux : Demux  Outputs=3
  Divide{,1..3} (4 alike) : Product  Inputs=*/
  Gain : Gain  Gain=-1
  Gain1 : Gain  Gain=-1
  Mux : Mux  Inputs=3
  Product{,3,8,11} (4 alike) : Product
  Product4 : Product  Inputs=3
  Product9 : Product  Inputs=3
  Sin : Trigonometry
  Sin1 : Trigonometry
  Sin2 : Trigonometry
  Sin3 : Trigonometry  Operator=cos
  Subtract1 : Sum  Inputs=--
  Subtract3 : Sum  Inputs=-+
  Out1 : Outport
  wires:
  Cos/1 -> [cosPhi313]
  Sin/1 -> [sinPhi313]
  Cos1/1 -> [cosTheta313]
  Demux/3 -> Sin2/1, Cos2/1
  Demux/1 -> Sin/1, Cos/1
  Sin2/1 -> [sinPsi313]
  Sin1/1 -> [sinTheta313]
  In1/1 -> Demux/1
  Demux/2 -> Sin1/1, Cos1/1
  Cos2/1 -> [cosPsi313]
  Mux/1 -> Out1/1
  [sinTheta312] -> Acos/1
  Atan3/1 -> Mux/3
  Atan2/1 -> Mux/1
  [sinPhi312] -> Atan2/1
  [cosPhi312] -> Atan2/2
  [sinPsi312] -> Atan3/1
  [cosPsi312] -> Atan3/2
  Acos/1 -> Mux/2
  [sinTheta313] -> Product/2
  Product/1 -> Acos1/1, [sinTheta312]
  Sin3/1 -> [cosTheta312]
  [cosPsi313] -> Product/1
  Acos1/1 -> Sin3/1
  Gain/1 -> [sinPhi312]
  Divide/1 -> Gain/1
  [cosTheta312] -> Divide/2
  Product3/1 -> Subtract1/1
  [cosPhi313] -> Product3/2
  Product4/1 -> Subtract1/2
  [cosPsi313] -> Product4/1
  [sinPhi313] -> Product4/2
  Subtract1/1 -> Divide/1
  [sinPsi313] -> Product3/1
  [cosTheta313] -> Product4/3
  [cosTheta312] -> Divide1/2
  Divide1/1 -> [cosPhi312]
  [cosPsi313] -> Product9/1
  Product9/1 -> Subtract3/2
  [sinPsi313] -> Product8/1
  [sinPhi313] -> Product8/2
  Product8/1 -> Subtract3/1
  [cosTheta313] -> Product9/3
  Subtract3/1 -> Divide1/1
  [cosPhi313] -> Product9/2
  Divide2/1 -> Gain1/1
  [cosTheta312] -> Divide2/2
  Gain1/1 -> [sinPsi312]
  [sinTheta313] -> Product11/2
  Product11/1 -> Divide2/1
  [sinPsi313] -> Product11/1
  [cosTheta312] -> Divide3/2
  [cosTheta313] -> Divide3/1
  Divide3/1 -> [cosPsi312]

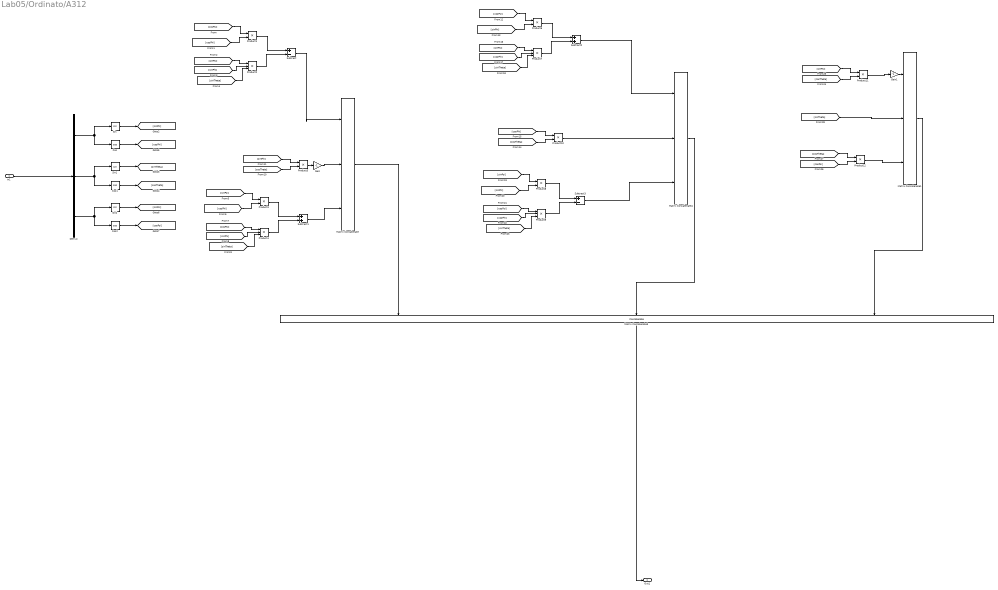
== system Lab05/Ordinato/A312 ==
  In1 : Inport
  Cos : Trigonometry  Operator=cos
  Cos1 : Trigonometry  Operator=cos
  Cos2 : Trigonometry  Operator=cos
  Demux : Demux  Outputs=3
  Gain : Gain  Gain=-1
  Gain1 : Gain  Gain=-1
  Matrix Concatenate : Concatenate  NumInputs=3  Mode=Multidimensional array
  Matrix Concatenate1 : Concatenate  NumInputs=3  Mode=Multidimensional array
  Matrix Concatenate3 : Concatenate  NumInputs=3  Mode=Multidimensional array  ConcatenateDimension=2
  Matrix Concatenate4 : Concatenate  NumInputs=3  Mode=Multidimensional array
  Product{1,3,5..6,8,10..12} (8 alike) : Product
  Product{2,4,7,9} (4 alike) : Product  Inputs=3
  Sin : Trigonometry
  Sin1 : Trigonometry
  Sin2 : Trigonometry
  Subtract : Sum  Inputs=+-
  Subtract1 : Sum
  Subtract2 : Sum
  Subtract3 : Sum  Inputs=+-
  Out1 : Outport
  wires:
  In1/1 -> Demux/1
  [sinTheta] -> Product2/3
  Product7/1 -> Subtract2/2
  [cosTheta] -> Product11/2
  [sinPhi] -> Product8/2
  Sin/1 -> [sinPhi]
  [sinPhi] -> Product2/2
  [cosTheta] -> Product10/2
  [cosPsi] -> Product6/1
  Demux/3 -> Sin2/1, Cos2/1
  Product9/1 -> Subtract3/2
  [sinTheta] -> Matrix Concatenate1/2
  Matrix Concatenate1/1 -> Matrix Concatenate3/3
  [sinPsi] -> Product11/1
  Product2/1 -> Subtract/2
  Subtract2/1 -> Matrix Concatenate4/1
  Matrix Concatenate4/1 -> Matrix Concatenate3/2
  [cosTheta] -> Product12/1
  Cos2/1 -> [cosPsi]
  [sinPsi] -> Product2/1
  [sinPsi] -> Product8/1
  Sin2/1 -> [sinPsi]
  [sinTheta] -> Product7/3
  Subtract/1 -> Matrix Concatenate/1
  [cosPhi] -> Product10/1
  Demux/2 -> Sin1/1, Cos1/1
  [sinTheta] -> Product9/3
  Product8/1 -> Subtract3/1
  [cosPhi] -> Product9/2
  [cosPsi] -> Product9/1
  Product11/1 -> Gain1/1
  Product1/1 -> Subtract/1
  [cosPhi] -> Product1/2
  [cosPsi] -> Product12/2
  [cosPhi] -> Product7/2
  [sinPhi] -> Product6/2
  Product6/1 -> Subtract2/1
  Demux/1 -> Sin/1, Cos/1
  [cosPsi] -> Product1/1
  [sinPsi] -> Product7/1
  Cos1/1 -> [cosTheta]
  Sin1/1 -> [sinTheta]
  Product12/1 -> Matrix Concatenate1/3
  Matrix Concatenate/1 -> Matrix Concatenate3/1
  Cos/1 -> [cosPhi]
  Matrix Concatenate3/1 -> Out1/1
  Gain1/1 -> Matrix Concatenate1/1
  Product10/1 -> Matrix Concatenate4/2
  Subtract3/1 -> Matrix Concatenate4/3
  [cosPsi] -> Product4/1
  Product4/1 -> Subtract1/2
  [cosPhi] -> Product3/2
  Product3/1 -> Subtract1/1
  [sinPsi] -> Product3/1
  [sinPhi] -> Product4/2
  [sinTheta] -> Product4/3
  [sinPhi] -> Product5/1
  [cosTheta] -> Product5/2
  Product5/1 -> Gain/1
  Subtract1/1 -> Matrix Concatenate/3
  Gain/1 -> Matrix Concatenate/2
